simulink model "DigitalInternalControl"  (R2015b)
settings: Solver=VariableStepAuto  StartTime=0.0  StopTime=500  RelTol=1e-3
settings Model: Creator=言厚  LastModifiedBy=言厚

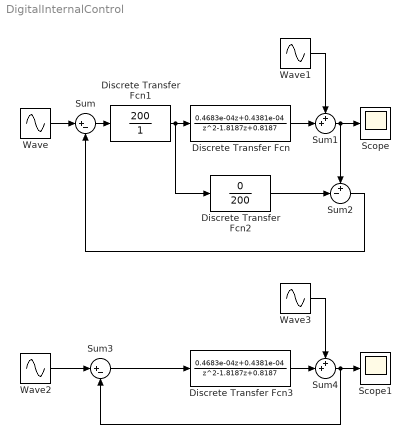
== system DigitalInternalControl ==
  Discrete Transfer Fcn : DiscreteTransferFcn  Numerator=[0.4683e-04 0.4381e-04]  Denominator="[1 -1.8187  0.8187]"
  Discrete Transfer Fcn1 : DiscreteTransferFcn  Numerator=[200]  Denominator=[1]
  Discrete Transfer Fcn2 : DiscreteTransferFcn  Numerator=[0]  Denominator=[200]
  Discrete Transfer Fcn3 : DiscreteTransferFcn  Numerator=[0.4683e-04 0.4381e-04]  Denominator="[1 -1.8187  0.8187]"
  Scope : Scope
  Scope1 : Scope
  Sum : Sum  Inputs=|+-
  Sum1 : Sum  Inputs=++|
  Sum2 : Sum  Inputs=+-|
  Sum3 : Sum  Inputs=|+-
  Sum4 : Sum  Inputs=++|
  Wave : Sin  SineType=Sample based  Amplitude=50  Samples=100  SampleTime=1
  Wave1 : Sin  SineType=Sample based  Amplitude=10  Bias=5  Samples=60  SampleTime=1
  Wave2 : Sin  SineType=Sample based  Amplitude=50  Samples=100  SampleTime=1
  Wave3 : Sin  SineType=Sample based  Amplitude=10  Bias=5  Samples=60  SampleTime=1
  wires:
  Wave/1 -> Sum/1
  Sum/1 -> Discrete Transfer Fcn1/1
  Discrete Transfer Fcn1/1 -> Discrete Transfer Fcn2/1, Discrete Transfer Fcn/1
  Sum1/1 -> Scope/1, Sum2/1
  Discrete Transfer Fcn2/1 -> Sum2/2
  Discrete Transfer Fcn/1 -> Sum1/2
  Sum2/1 -> Sum/2
  Wave1/1 -> Sum1/1
  Wave2/1 -> Sum3/1
  Discrete Transfer Fcn3/1 -> Sum4/2
  Sum4/1 -> Scope1/1, Sum3/2
  Wave3/1 -> Sum4/1
  Sum3/1 -> Discrete Transfer Fcn3/1
